simulink model "advanced_system_model"  (R2025b)
settings: Solver=VariableStepAuto  StartTime=0.0  StopTime=10.0  RelTol=1e-3
values from neighbouring files (symbols this model uses):
  A = 1    [system_variables.m]
  a = 1    [system_variables.m]
  p = 1    [system_variables.m]
  T = 1    [system_variables.m]
libraries: simulink x1
settings Model: Creator=techn  LastModifiedBy=YSFADE001

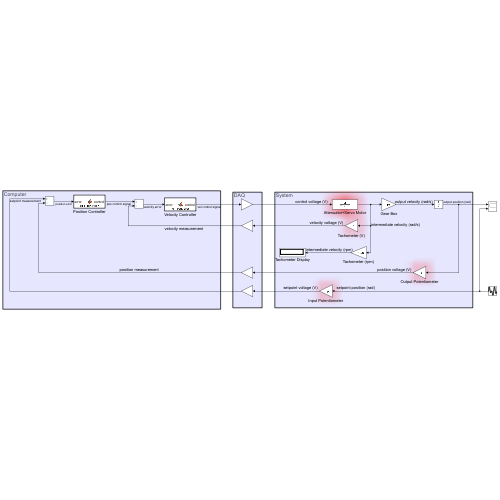
[thumbnail: Simulink's stored preview of the top-level diagram]
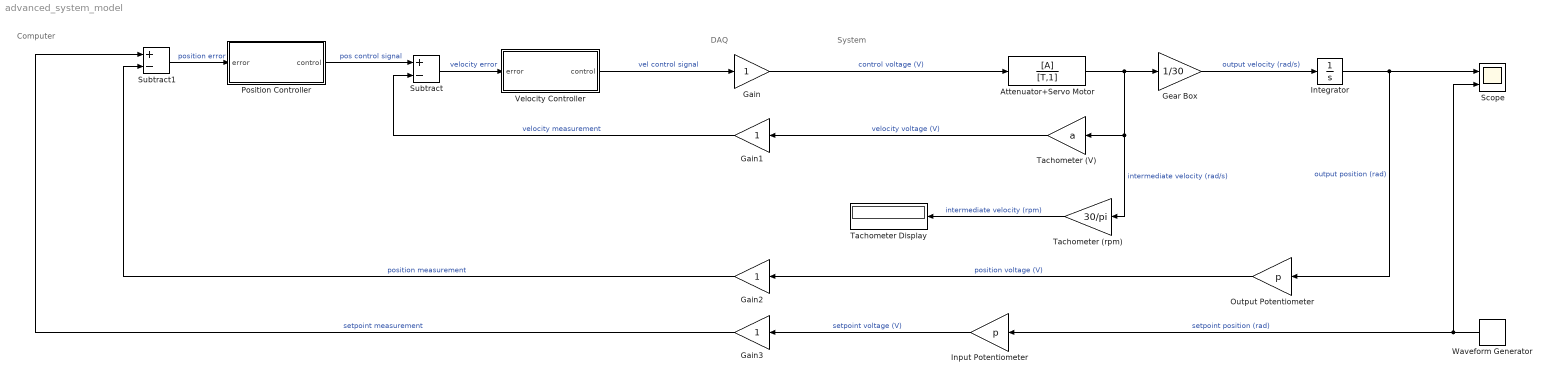
== system advanced_system_model ==
  note: System
  note: Computer
  note: DAQ
  Attenuator+Servo Motor : TransferFcn  Numerator=[A]  Denominator=[T,1]
  Gain{,1..3} (4 alike) : Gain
  Gear Box : Gain  Gain=1/30
  Input Potentiometer : Gain  Gain=p
  Integrator : Integrator
  Output Potentiometer : Gain  Gain=p
  Position Controller : MATLAB Function  TreatAsAtomicUnit=on
  Scope : Scope  NumInputPorts=2
  Subtract : Sum  Inputs=+-
  Subtract1 : Sum  Inputs=+-
  Tachometer (V) : Gain  Gain=a
  Tachometer (rpm) : Gain  Gain=30/pi
  Tachometer Display : Display
  Velocity Controller : MATLAB Function  TreatAsAtomicUnit=on
  Waveform Generator : simulink/Sources/Waveform Generator  OutMin=[]  OutMax=[]  OutDataTypeStr=double  SelectedSignal=1  BlockNames=MultiportSwitch_e3df3653d217406  SampleTime=0.1
  wires:
  Attenuator+Servo Motor/1 -> Tachometer (V)/1, Tachometer (rpm)/1, Gear Box/1  "intermediate velocity (rad/s)"
  Gear Box/1 -> Integrator/1  "output velocity (rad/s)"
  Tachometer (rpm)/1 -> Tachometer Display/1  "intermediate velocity (rpm)"
  Integrator/1 -> Scope/1, Output Potentiometer/1  "output position (rad)"
  Waveform Generator/1 -> Input Potentiometer/1, Scope/2  "setpoint position (rad)"
  Input Potentiometer/1 -> Gain3/1  "setpoint voltage (V)"
  Gain/1 -> Attenuator+Servo Motor/1  "control voltage (V)"
  Tachometer (V)/1 -> Gain1/1  "velocity voltage (V)"
  Output Potentiometer/1 -> Gain2/1  "position voltage (V)"
  Velocity Controller/1(control) -> Gain/1  "vel control signal"
  Subtract/1 -> Velocity Controller/1(error)  "velocity error"
  Position Controller/1(control) -> Subtract/1  "pos control signal"
  Subtract1/1 -> Position Controller/1(error)  "position error"
  Gain3/1 -> Subtract1/1  "setpoint measurement"
  Gain1/1 -> Subtract/2  "velocity measurement"
  Gain2/1 -> Subtract1/2  "position measurement"

== matlab function advanced_system_model/Velocity Controller ==
  data: error input; control output
function control = vel_controller(error)
    control = error;
end

== matlab function advanced_system_model/Position Controller ==
  data: error input; control output
function control = pos_controller(error)
    control = error;
end
